simulink model "salimbtp"  (R2023b)
settings: Solver=VariableStepAuto  StartTime=0.0  StopTime=10.0  RelTol=1e-3
settings Model: Creator=Dell  LastModifiedBy=Dell

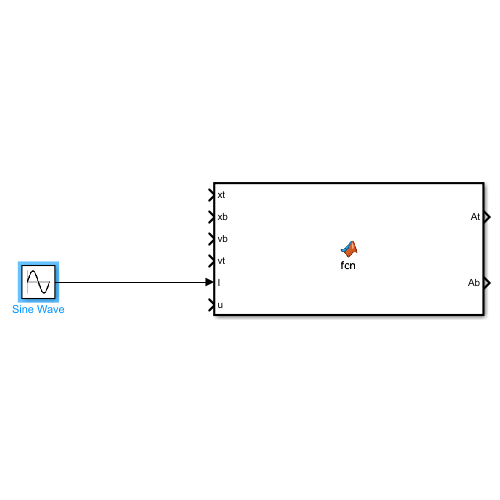
[thumbnail: Simulink's stored preview of the top-level diagram]
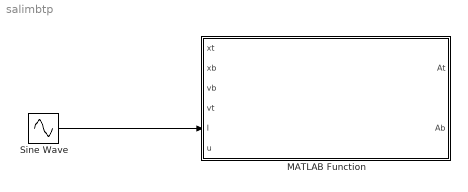
== system salimbtp ==
  MATLAB Function : MATLAB Function  TreatAsAtomicUnit=on
  Sine Wave : Sin  SampleTime=0
  wires:
  Sine Wave/1 -> MATLAB Function/5(I)

== matlab function salimbtp/MATLAB Function ==
  data: xt input; At output; xb input; vb input; vt input; I input; Ab output; u input
function [At, Ab]= fcn(xt,xb,vb, vt, I, u)

    Mt = 10.06;
    Kt = 9582;
    bl = 6.114;
    Mb = 3.24;
    Ct = 12.36;
    Cb = 153.0096;
    Kb = 89140.8;
    L  = 74.8*10^-6;
    R  = 1.34;
    
    Ebemf = 6.096*(vt-vb);
    Iprime = (u-I*R -Ebemf)/L;

    At =-(bl*I + Kt(xt-xb) + Ct(vt-vb))/ Mt;

    Ab =-(bl*I - Kt(xt-xb) - Ct(vt-vb) +Kb*xb +Cb*vb)/ Mb;
